simulink model "tempControlEmbedded"  (R2013b)
settings: Solver=ode3  SolverMode=SingleTasking  StartTime=0.0  StopTime=inf  RelTol=1e-3
libraries: arduinolib x2
settings Model: ExtModeTrigDuration=2  Creator=gcampa  LastModifiedBy=richard.hill
settings OptimizationCC: OptimizeModelRefInitCode=on  LifeSpan=1
settings DebuggingCC: SolverPrmCheckMsg=none
settings HardwareCC: ProdBitPerInt=16  ProdBitPerPointer=8  ProdIntDivRoundTo=Zero  ProdEndianess=LittleEndian  ProdWordSize=8  ProdHWDeviceType=Atmel->AVR
settings RTWCC: SystemTargetFile=realtime.tlc  GenerateMakefile=off  TemplateMakefile=realtime.tmf  Description=Run on Target Hardware  RTWVerbose=off  ProcessScript=realtime_make_rtw_hook
settings STFCustomTargetCC: TargetLibSuffix=.a  GenerateSampleERTMain=on  ERTCustomFileBanners=on  SupportNonInlinedSFcns=off  SupportVariableSizeSignals=on  MATLABClassNameForMDSCustomization=Simulink.SoftwareTarget.ERTCustomization  GRTInterface=off  SystemTargetFile=realtime.tlc
settings ERTTargetCC: CodeReplacementLibrary=ANSI_C  GenerateSampleERTMain=on  ParMdlRefBuildCompliant=off  CompOptLevelCompliant=off  ConcurrentExecutionCompliant=off  CombineOutputUpdateFcns=off  ERTFirstTimeCompliant=off  SupportContinuousTime=on  SupportVariableSizeSignals=on  ModelStepFunctionPrototypeControlCompliant=off  CPPClassGenCompliant=off  ExtModeTransport=3  ExtModeMexFile=ext_serial_win32_comm  ExtModeMexArgs=0 1 9600  InlinedParameterPlacement=NonHierarchical  ERTSrcFileBannerTemplate=realtime_code_template.cgt  ERTHdrFileBannerTemplate=realtime_code_template.cgt  ERTDataSrcFileTemplate=realtime_code_template.cgt  ERTDataHdrFileTemplate=realtime_code_template.cgt  ERTCustomFileTemplate=realtime_file_process.tlc

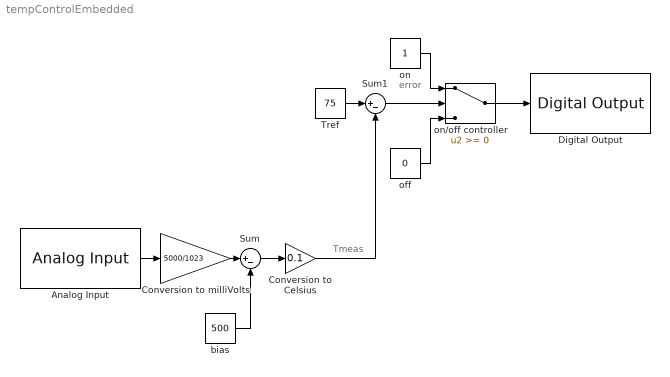
== system tempControlEmbedded ==
  note: error
  note: Tmeas
  Analog Input : arduinolib/Analog Input  pinNumber=0  sampleTime=0.1
  Conversion to Celsius : Gain  Gain=0.1
  Conversion to milliVolts : Gain  Gain=5000/1023
  Digital Output : arduinolib/Digital Output  pinNumber=9
  Sum : Sum  Inputs=|+-
  Sum1 : Sum  Inputs=|+-
  Tref : Constant  Value=75
  bias : Constant  Value=500
  off : Constant  Value=0
  on : Constant
  on/off controller : Switch
  wires:
  Analog Input/1 -> Conversion to milliVolts/1
  Conversion to milliVolts/1 -> Sum/1
  on/off controller/1 -> Digital Output/1
  Sum/1 -> Conversion to Celsius/1
  bias/1 -> Sum/2
  Tref/1 -> Sum1/1
  Sum1/1 -> on/off controller/2
  on/1 -> on/off controller/1
  off/1 -> on/off controller/3
  Conversion to Celsius/1 -> Sum1/2
